simulink model "HighlyDynamicTrajectory_EuroGNC2022"  (R2018b)
settings: Solver=ode4  StartTime=0.0  StopTime=43.381  FixedStep=0.001  RelTol=1e-3
values from neighbouring files (symbols this model uses):
  airplane = conventionalAirplaneLoadParams(  	'params_conventional_airplane_EasyGlider' )    [init_HighlyDynamicTrajectory_EuroGNC2022.m]
  envir = envirLoadParams( 'envir_params_default', 'envir', 0 )    [init_HighlyDynamicTrajectory_EuroGNC2022.m]
  g = 9.81    [init_HighlyDynamicTrajectory_EuroGNC2022.m]
  inital_vel_vec = inital_velo * T    [init_HighlyDynamicTrajectory_EuroGNC2022.m]
  K_atti = ndiFeedbackGainPlace( -10*ones(3,1), 2/80 + 2/100 )    [init_HighlyDynamicTrajectory_EuroGNC2022.m]
  K_lateral = ndiFeedbackGainPlace( -0.75*ones(3,1), 0)    [init_HighlyDynamicTrajectory_EuroGNC2022.m]
  K_vertical = ndiFeedbackGainPlace(-2.0*ones(3,1), 0)    [init_HighlyDynamicTrajectory_EuroGNC2022.m]
  traj = trajFromWaypoints(traj, waypoints, degree, cycle)    [init_HighlyDynamicTrajectory_EuroGNC2022.m]
undefined symbols (not defined in the file or in its folder): aileron_left, aileron_right, alt_ground, atmosphere, ca, elevator, htp_trim, rudder, throttle, wind
libraries: actuators_lib x7, simulink x7, unit_conversions_lib x7, axes_transformation_lib x1, quat_lib x1, indi_lib x1, quatAttitudeController_lib x1, conventional_airplane_single_engine_lib x1, atmosphere_lib x1, sensors_lib x1, flightgear_visualization_lib x1
settings Model: Creator=Fgücker  LastModifiedBy=fabian

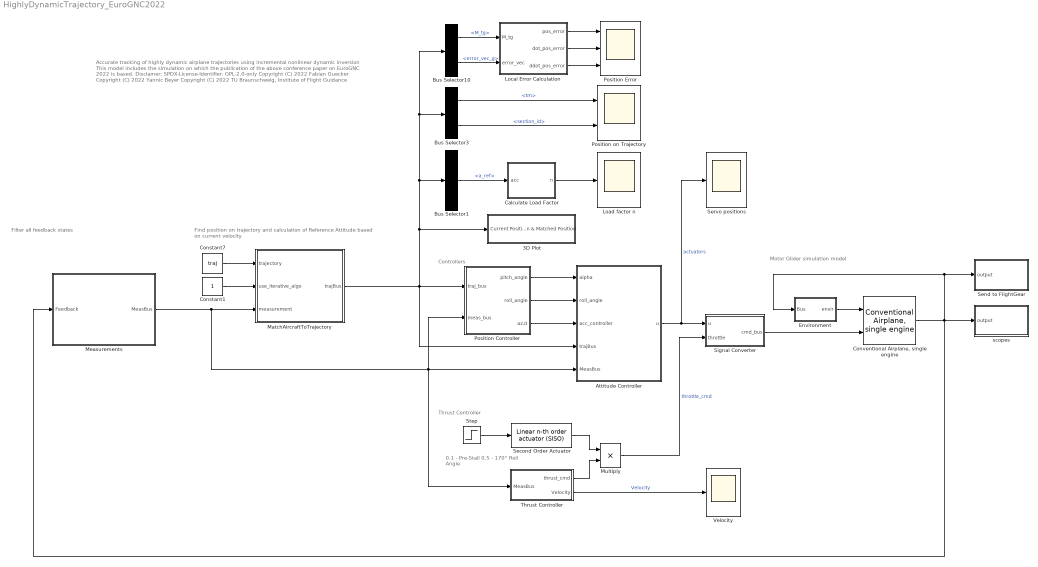
== system HighlyDynamicTrajectory_EuroGNC2022 ==
  note: Controllers
  note: 0.1 - Pre-Stall
      | 0.5 - 170° Roll Angle
  note: Accurate tracking of highly dynamic airplane
      | trajectories using incremental nonlinear dynamic
      | inversion
      |
      | This model includes the simulation on which the publication of the above conference paper on EuroGNC 2022 is based.
      |
      | Disclamer:
      | SPDX-License-Identifier: GPL-2.0-only
      |
      | Copyright (C) 2022 Fabian Guecker
      | Copyright (C) 2022 Yannic Beyer
      | Copyright (C) 2022 TU Braunschweig, Institute of Flight Guidance
  note: Thrust Controller
  note: Find position on trajectory and calculation
      | of Reference Attitude based on current velocity
  note: Filter all feedback states
  note: Motor Glider simulation model
  3D Plot : Subsystem
  Attitude Controller : Subsystem
  Bus Selector1 : BusSelector  OutputSignals=a_ref
  Bus Selector10 : BusSelector  OutputSignals=M_tg,error_vec_g
  Bus Selector3 : BusSelector  OutputSignals=tm,section_id
  Calculate Load Factor : Subsystem
  Constant1 : Constant
  Constant7 : Constant  Value=traj  OutDataTypeStr=Bus: trajectoryBus
  "Conventional Airplane, single engine" : conventional_airplane_single_engine_lib/Conventional Airplane, single engine  airplane=airplane
      settings: SourceProductName=LADAC
  Environment : Subsystem
  Load factor n : Scope
  Local Error Calculation : Subsystem
  MatchAircraftToTrajectory : Subsystem  SystemSampleTime=0.001
  Measurements : Subsystem  mask{omega0=50, D=0.55}
      mask prompts: omega0 "Omega - Filter"; D "Damping D - Filter"
  Multiply : Product
  Position Controller : Subsystem
  Position Error : Scope  NumInputPorts=3
  Position on Trajectory : Scope  NumInputPorts=2
  Second Order Actuator : actuators_lib/Linear n-th order actuator (SISO)  omega=10  order=2  output_order=1  use_inital_value=on
      settings: SourceProductName=LADAC
  Send to FlightGear : Subsystem
  Servo positions : Scope
  Signal Converter : Subsystem
  Step : Step  Time=26  Before=0.1  After=0.5  SampleTime=0
  Thrust Controller : Subsystem
  Velocity : Scope
  scopes : Subsystem
  wires:
  Measurements/1(MeasBus) -> Attitude Controller/5(MeasBus), Thrust Controller/1(MeasBus), Position Controller/2(meas_bus), MatchAircraftToTrajectory/3(measurement)
  Thrust Controller/1(thrust_cmd) -> Multiply/2
  Thrust Controller/2(Velocity) -> Velocity/1  "Velocity"
  Environment/1(envir) -> "Conventional Airplane, single engine"/1
  Local Error Calculation/3(ddot_pos_error) -> Position Error/3
  Local Error Calculation/2(dot_pos_error) -> Position Error/2
  Local Error Calculation/1(pos_error) -> Position Error/1
  Bus Selector10/2 -> Local Error Calculation/2(error_vec)  "<error_vec_g>"
  Multiply/1 -> Signal Converter/2(throttle)  "throttle_cmd"
  Constant7/1 -> MatchAircraftToTrajectory/1(trajectory)
  Bus Selector10/1 -> Local Error Calculation/1(M_tg)  "<M_tg>"
  Calculate Load Factor/1(n) -> Load factor n/1
  Bus Selector1/1 -> Calculate Load Factor/1(acc)  "<a_ref>"
  Bus Selector3/1 -> Position on Trajectory/1  "<tm>"
  Bus Selector3/2 -> Position on Trajectory/2  "<section_id>"
  Position Controller/1(pitch_angle) -> Attitude Controller/1(alpha)
  Position Controller/2(roll_angle) -> Attitude Controller/2(roll_angle)
  Constant1/1 -> MatchAircraftToTrajectory/2(use_iterative_algo)
  Position Controller/3(az,d) -> Attitude Controller/3(acc_controller)
  Step/1 -> Second Order Actuator/1
  Second Order Actuator/1 -> Multiply/1
  Signal Converter/1(cmd_bus) -> "Conventional Airplane, single engine"/2
  Attitude Controller/1(u) -> Servo positions/1, Signal Converter/1(u)  "actuators"
  MatchAircraftToTrajectory/1(trajBus) -> Bus Selector1/1, Bus Selector10/1, Bus Selector3/1, 3D Plot/1(Current Position & Matched Position), Position Controller/1(traj_bus), Attitude Controller/4(trajBus)
  "Conventional Airplane, single engine"/1 -> Measurements/1(Feedback), Environment/1(Bus), Send to FlightGear/1(output), scopes/1(output)

== system HighlyDynamicTrajectory_EuroGNC2022/3D Plot ==
  Current Position & Matched Position : Inport
  3D Graph : S-Function  LoadFcn=if exist('sfun3d','file'), sfun3d([],[],[],'LoadBlock'); end  FunctionName=sfun3d  Parameters=ax,T,np,cp,gd,ls,mk,mx,hd,tb  SFunctionDeploymentMode=off  EnableBusSupport=off  mask(3D Graph){np=2, ax=[-8 8 -8 8 -8 8]*20, mx=1e4, T=0.040, cp=[-1 -1 1]*35, gd=on, hd=off, tb=off, ls=-, mk=none}
      mask prompts: np "Number of moving points (lines)"; ax "Range: [xmin xmax  ymin ymax zmin zmax]"; mx "Max number of points in each line"; T "Sampling Time"; cp "Camera position (use [0 0 1] for 2D XY view)"; gd "Grid (on|off)"; hd "HeadMarkers (on|off)"; tb "Toolbar (on|off)"; ls "LineStyle"; mk "LineMarker"
      mask help:
      | This block plots the position of several points in the XYZ space. The input contains the coordinates of all the points (x1,y1,z1,x2,y2,z2,...).
      | The number of moving points (lines), the XYZ ranges, sampling time, camera position, and grid (among other things) can be set as mask parameters.
      settings: CopyFcn=if exist('sfun3d','file'), sfun3d([],[],[],'CopyBlock'); end  DeleteFcn=if exist('sfun3d','file'), sfun3d([],[],[],'DeleteBlock'); end  NameChangeFcn=if exist('sfun3d','file'), sfun3d([],[],[],'NameChange'); end
      mask Help:
      | This block plots the position of several points in the XYZ space. The input contains the coordinates of all the points (x1,y1,z1,x2,y2,z2,...).
      | The number of moving points (lines), the XYZ ranges, sampling time, camera position, and grid (among other things) can be set as mask parameters.
      mask TypeOptions ls: - | -- | : | -. | none
      mask TypeOptions mk: none | . | + | o | * | x | square | diamond | v | ^ | > | < | pentagram | hexagram
      mask Display: plot([.05 .95 .95 .05 .05],[.45 .45 .95 .95 .45], 0.5+cos(0:0.1:2*pi)*0.3,0.7+sin(0:0.1:2*pi)*0.2)
  Bus Selector5 : BusSelector  OutputSignals=s_g,position
  Gain19 : Gain  Gain=[1 1 -1]'
  Gain2 : Gain  Gain=[1 1 -1]'
  Mux : Mux  Inputs=2
  wires:
  Bus Selector5/2 -> Gain19/1  "<position>"
  Gain19/1 -> Mux/2
  Current Position & Matched Position/1 -> Bus Selector5/1
  Bus Selector5/1 -> Gain2/1  "<s_g>"
  Mux/1 -> 3D Graph/1
  Gain2/1 -> Mux/1

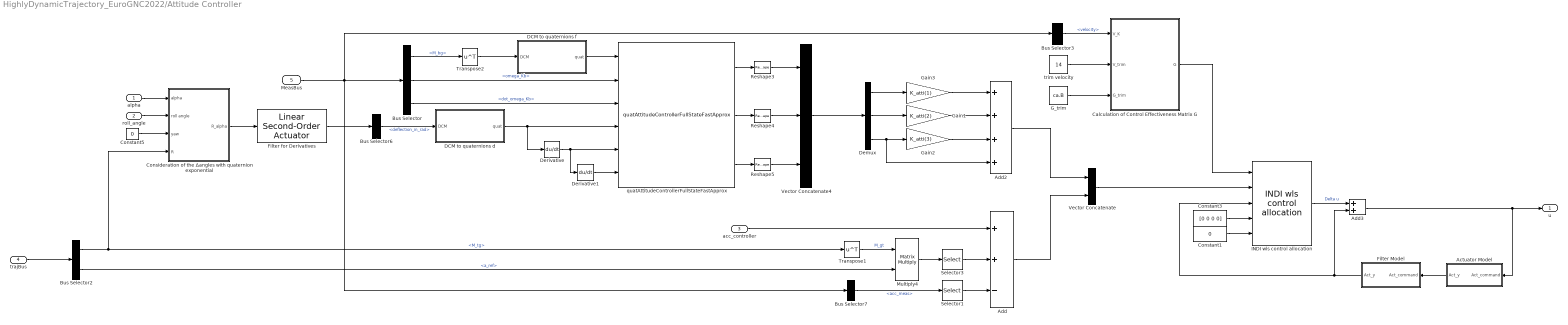
== system HighlyDynamicTrajectory_EuroGNC2022/Attitude Controller ==
  alpha : Inport
  roll_angle : Inport  Port=2
  acc_controller : Inport  Port=3
  trajBus : Inport  Port=4
  MeasBus : Inport  Port=5
  Actuator Model : Subsystem  mask{omega=[80 80 80 80]', d=1, A_0=[0 0 0 0]', dot_A_0=0, start_steady_state=off}
      mask prompts: omega "Natural frequency"; d "Damping ratio"; A_0 "Initial position"; dot_A_0 "Initial velocity"; start_steady_state "Start steady state"
  Add : Sum  Inputs=++-
  Add2 : Sum  Inputs=++++
  Add3 : Sum
  Bus Selector : BusSelector  OutputSignals=EKF.M_bg,EKF.omega_Kb,EKF.dot_omega_Kb
  Bus Selector2 : BusSelector  OutputSignals=M_tg,a_ref
  Bus Selector3 : BusSelector  OutputSignals=EKF.velocity
  Bus Selector6 : BusSelector  OutputSignals=deflection_in_rad
  Bus Selector7 : BusSelector  OutputSignals=accelerometer.acc_meas
  Calculation of Control Effectiveness Matrix G : Subsystem
  Consideration of the Δangles with quaternion exponential : Subsystem
  Constant1 : Constant  Value=0
  Constant3 : Constant  Value=[0 0 0 0]
  Constant5 : Constant  Value=0
  DCM to quaternions d : Subsystem
      mask DialogControl DescGroupVar Prompt: Get quaternions from DCM without discontinuities
      mask DialogControl DescTextVar Prompt: Look inside the block (and function) for more information.
  DCM to quaternions f : Subsystem
      mask DialogControl DescGroupVar Prompt: Get quaternions from DCM without discontinuities
      mask DialogControl DescTextVar Prompt: Look inside the block (and function) for more information.
  Demux : Demux  Outputs=3
  Derivative : Derivative
  Derivative1 : Derivative
  Filter Model : Subsystem  mask{omega=[50 50 50 50]', d=0.55, A_0=[0 0 0 0]', dot_A_0=0, start_steady_state=off}
      mask prompts: omega "Natural frequency"; d "Damping ratio"; A_0 "Initial position"; dot_A_0 "Initial velocity"; start_steady_state "Start steady state"
  Filter for Derivatives : actuators_lib/Linear Second-Order Actuator  omega=200  d=1  A_0=0  dot_A_0=0  start_steady_state=on
      settings: SourceProductName=LADAC
  G_trim : Constant  Value=ca.B
  Gain1 : Gain  Gain=K_atti(2)
  Gain2 : Gain  Gain=K_atti(3)
  Gain3 : Gain  Gain=K_atti(1)
  INDI wls control allocation : indi_lib/INDI wls control allocation  ca=ca
      settings: SourceProductName=LADAC
  Multiply4 : Product  Multiplication=Matrix(*)
  Reshape3 : Reshape  OutputDimensionality=Column vector (2-D)
  Reshape4 : Reshape  OutputDimensionality=Column vector (2-D)
  Reshape5 : Reshape  OutputDimensionality=Column vector (2-D)
  Selector1 : Selector  InputPortWidth=3  IndexOptions=Index vector (dialog)  Indices=[3]  OutputSizes=1
  Selector3 : Selector  InputPortWidth=3  IndexOptions=Index vector (dialog)  Indices=[3]  OutputSizes=1
  Transpose1 : Math  Operator=transpose  SaturateOnIntegerOverflow=on
  Transpose2 : Math  Operator=transpose  SaturateOnIntegerOverflow=on
  Vector Concatenate : Concatenate
  Vector Concatenate4 : Concatenate  NumInputs=3
  quatAttitudeControllerFullStateFastApprox : quatAttitudeController_lib/quatAttitudeControllerFullStateFastApprox  SystemSampleTime=-1
      settings: SourceProductName=LADAC
  trim velocity : Constant  Value=14
  u : Outport
  wires:
  Bus Selector/3 -> quatAttitudeControllerFullStateFastApprox/3  "<dot_omega_Kb>"
  Derivative1/1 -> quatAttitudeControllerFullStateFastApprox/6
  Filter for Derivatives/1 -> Bus Selector6/1
  Vector Concatenate4/1 -> Demux/1
  Bus Selector/2 -> quatAttitudeControllerFullStateFastApprox/2  "<omega_Kb>"
  Gain3/1 -> Add2/1
  Derivative/1 -> Derivative1/1, quatAttitudeControllerFullStateFastApprox/5
  Gain1/1 -> Add2/2
  Demux/3 -> Add2/4, Gain2/1
  Bus Selector/1 -> Transpose2/1  "<M_bg>"
  DCM to quaternions f/1(quat) -> quatAttitudeControllerFullStateFastApprox/1
  quatAttitudeControllerFullStateFastApprox/1 -> Reshape3/1
  Reshape3/1 -> Vector Concatenate4/1
  Reshape4/1 -> Vector Concatenate4/2
  Reshape5/1 -> Vector Concatenate4/3
  quatAttitudeControllerFullStateFastApprox/3 -> Reshape5/1
  Bus Selector6/1 -> DCM to quaternions d/1(DCM)  "<deflection_in_rad>"
  quatAttitudeControllerFullStateFastApprox/2 -> Reshape4/1
  roll_angle/1 -> Consideration of the Δangles with quaternion exponential/2(roll angle)
  Demux/1 -> Gain3/1
  Gain2/1 -> Add2/3
  Demux/2 -> Gain1/1
  DCM to quaternions d/1(quat) -> Derivative/1, quatAttitudeControllerFullStateFastApprox/4
  Transpose2/1 -> DCM to quaternions f/1(DCM)
  INDI wls control allocation/1 -> Add3/1  "Delta u"
  Bus Selector7/1 -> Selector1/1  "<acc_meas>"
  Transpose1/1 -> Multiply4/1  "M_gt"
  trajBus/1 -> Bus Selector2/1
  Multiply4/1 -> Selector3/1
  Bus Selector2/2 -> Multiply4/2  "<a_ref>"
  Selector1/1 -> Add/3
  Bus Selector2/1 -> Consideration of the Δangles with quaternion exponential/4(R), Transpose1/1  "<M_tg>"
  Vector Concatenate/1 -> INDI wls control allocation/2
  Add/1 -> Vector Concatenate/2
  acc_controller/1 -> Add/1
  Selector3/1 -> Add/2
  Add3/1 -> u/1, Actuator Model/1(Act_command)
  alpha/1 -> Consideration of the Δangles with quaternion exponential/1(alpha)
  MeasBus/1 -> Bus Selector3/1, Bus Selector7/1, Bus Selector/1
  Constant3/1 -> INDI wls control allocation/4
  Consideration of the Δangles with quaternion exponential/1(R_alpha) -> Filter for Derivatives/1
  Constant5/1 -> Consideration of the Δangles with quaternion exponential/3(yaw)
  Filter Model/1(Act_y) -> Add3/2, INDI wls control allocation/3
  Actuator Model/1(Act_y) -> Filter Model/1(Act_command)
  Bus Selector3/1 -> Calculation of Control Effectiveness Matrix G/1(V_K)  "<velocity>"
  trim velocity/1 -> Calculation of Control Effectiveness Matrix G/2(V_trim)
  G_trim/1 -> Calculation of Control Effectiveness Matrix G/3(G_trim)
  Calculation of Control Effectiveness Matrix G/1(G) -> INDI wls control allocation/1
  Constant1/1 -> INDI wls control allocation/5
  Add2/1 -> Vector Concatenate/1

== system HighlyDynamicTrajectory_EuroGNC2022/Calculate Load Factor ==
  acc : Inport
  Dot Product : DotProduct  InputSameDT=on  OutDataTypeStr=Inherit: Inherit via internal rule
  Gain7 : Gain  Gain=1/g
  Sqrt : Sqrt  SaturateOnIntegerOverflow=on
  n : Outport
  wires:
  Dot Product/1 -> Sqrt/1
  Sqrt/1 -> Gain7/1
  acc/1 -> Dot Product/1, Dot Product/2
  Gain7/1 -> n/1

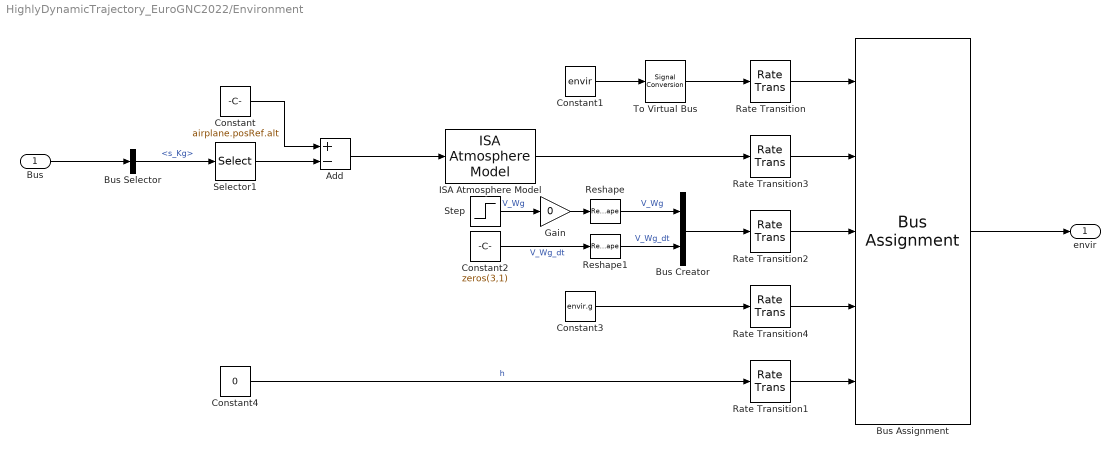
== system HighlyDynamicTrajectory_EuroGNC2022/Environment ==
  Bus : Inport
  Add : Sum  Inputs=+-
  Bus Assignment : BusAssignment  AssignedSignals=atmosphere,wind,g,alt_ground
  Bus Creator : BusCreator  Inputs=2
  Bus Selector : BusSelector  OutputSignals=rigidBodyBus.s_Kg
  Constant : Constant  Value=airplane.posRef.alt
  Constant1 : Constant  Value=envir  OutDataTypeStr=Bus: envirBus
  Constant2 : Constant  Value=zeros(3,1)
  Constant3 : Constant  Value=envir.g
  Constant4 : Constant  Value=0
  Gain : Gain  Gain=0
  ISA Atmosphere Model : atmosphere_lib/ISA Atmosphere Model  SystemSampleTime=-1
      settings: SourceProductName=LADAC
  Rate Transition{,1..4} (5 alike) : RateTransition
  Reshape : Reshape  OutputDimensionality=Column vector (2-D)
  Reshape1 : Reshape  OutputDimensionality=Column vector (2-D)
  Selector1 : Selector  InputPortWidth=3  IndexOptions=Index vector (dialog)  Indices=3  OutputSizes=1
  Step : Step  Time=3  After=[0;5;0]  SampleTime=0
  To Virtual Bus : SignalConversion  ConversionOutput=Virtual bus  OverrideOpt=off
  envir : Outport
  wires:
  Constant4/1 -> Rate Transition1/1  "h"
  Rate Transition2/1 -> Bus Assignment/3
  Rate Transition3/1 -> Bus Assignment/2
  Bus Assignment/1 -> envir/1
  Rate Transition/1 -> Bus Assignment/1
  ISA Atmosphere Model/1 -> Rate Transition3/1
  Step/1 -> Gain/1  "V_Wg"
  Rate Transition1/1 -> Bus Assignment/5
  Constant1/1 -> To Virtual Bus/1
  Bus/1 -> Bus Selector/1
  Bus Creator/1 -> Rate Transition2/1
  Constant2/1 -> Reshape1/1  "V_Wg_dt"
  Rate Transition4/1 -> Bus Assignment/4
  Constant3/1 -> Rate Transition4/1
  Gain/1 -> Reshape/1
  Constant/1 -> Add/1
  Add/1 -> ISA Atmosphere Model/1
  Selector1/1 -> Add/2
  To Virtual Bus/1 -> Rate Transition/1
  Reshape/1 -> Bus Creator/1  "V_Wg"
  Reshape1/1 -> Bus Creator/2  "V_Wg_dt"
  Bus Selector/1 -> Selector1/1  "<s_Kg>"

== system HighlyDynamicTrajectory_EuroGNC2022/Local Error Calculation ==
  M_tg : Inport
  error_vec : Inport  Port=2
  Derivative1 : Derivative
  Derivative2 : Derivative
  Multiply2 : Product  Multiplication=Matrix(*)
  Transpose : Math  Operator=transpose  SaturateOnIntegerOverflow=on
  pos_error : Outport
  dot_pos_error : Outport  Port=2
  ddot_pos_error : Outport  Port=3
  wires:
  error_vec/1 -> Multiply2/2
  Transpose/1 -> Multiply2/1
  M_tg/1 -> Transpose/1
  Derivative1/1 -> dot_pos_error/1, Derivative2/1
  Derivative2/1 -> ddot_pos_error/1
  Multiply2/1 -> Derivative1/1, pos_error/1

== system HighlyDynamicTrajectory_EuroGNC2022/MatchAircraftToTrajectory ==
  trajectory : Inport
  use_iterative_algo : Inport  Port=2
  measurement : Inport  Port=3
  Bus Creator : BusCreator  Inputs=8
  Bus Selector1 : BusSelector  OutputSignals=EKF.s_g,EKF.velocity
  Bus Selector3 : BusSelector  OutputSignals=EKF.s_g,EKF.velocity
  Constant : Constant  Value=[0; 0; -g]  VectorParams1D=off
  MATLAB Function6 : MATLAB Function  TreatAsAtomicUnit=on
  trajBus : Outport
  wires:
  Bus Selector3/1 -> MATLAB Function6/2(pos_ac)  "<s_g>"
  trajectory/1 -> MATLAB Function6/1(traj)  "trajectory"
  measurement/1 -> Bus Selector1/1, Bus Selector3/1
  Bus Creator/1 -> trajBus/1
  Bus Selector3/2 -> MATLAB Function6/3(vel)  "<velocity>"
  Constant/1 -> MATLAB Function6/4(acc_vec)
  use_iterative_algo/1 -> MATLAB Function6/5(use_iterative_algo)
  MATLAB Function6/1(pos) -> Bus Creator/1  "position"
  MATLAB Function6/2(error_vec) -> Bus Creator/2  "error_vec_g"
  MATLAB Function6/3(section_idx) -> Bus Creator/3  "section_id"
  MATLAB Function6/4(t) -> Bus Creator/4  "tm"
  MATLAB Function6/5(a_ref) -> Bus Creator/5  "a_ref"
  MATLAB Function6/6(M_tg) -> Bus Creator/6  "M_tg"
  Bus Selector1/1 -> Bus Creator/7  "<s_g>"
  Bus Selector1/2 -> Bus Creator/8  "<velocity>"

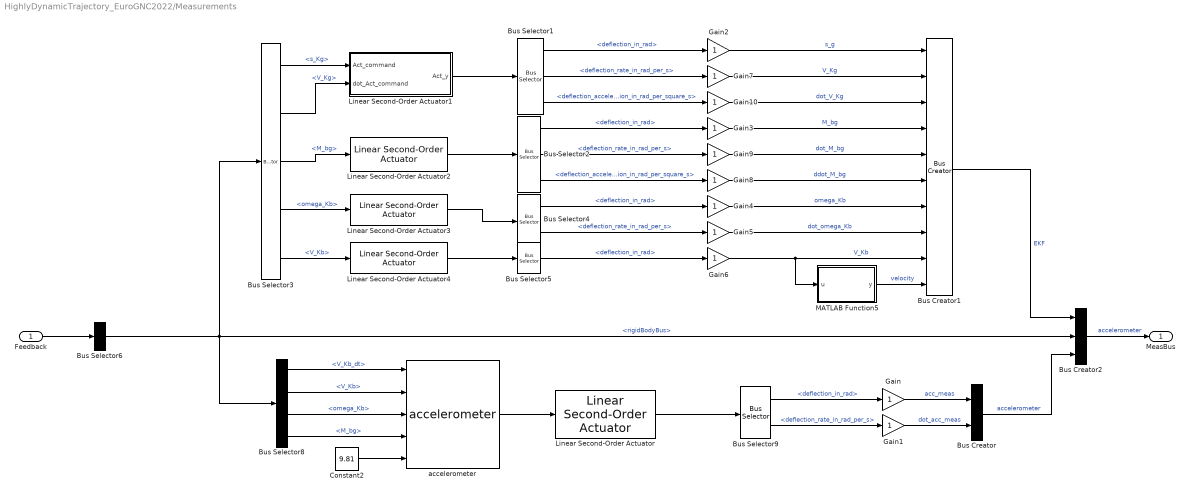
== system HighlyDynamicTrajectory_EuroGNC2022/Measurements ==
  Feedback : Inport
  Bus Creator : BusCreator  Inputs=2
  Bus Creator1 : BusCreator  Inputs=10
  Bus Creator2 : BusCreator  Inputs=3
  Bus Selector1 : BusSelector  OutputSignals=deflection_in_rad,deflection_rate_in_rad_per_s,deflection_acceleration_in_rad_per_square_s
  Bus Selector2 : BusSelector  OutputSignals=deflection_in_rad,deflection_rate_in_rad_per_s,deflection_acceleration_in_rad_per_square_s
  Bus Selector3 : BusSelector  OutputSignals=s_Kg,V_Kg,M_bg,omega_Kb,V_Kb
  Bus Selector4 : BusSelector  OutputSignals=deflection_in_rad,deflection_rate_in_rad_per_s
  Bus Selector5 : BusSelector  OutputSignals=deflection_in_rad
  Bus Selector6 : BusSelector  OutputSignals=rigidBodyBus
  Bus Selector8 : BusSelector  OutputSignals=V_Kb_dt,V_Kb,omega_Kb,M_bg
  Bus Selector9 : BusSelector  OutputSignals=deflection_in_rad,deflection_rate_in_rad_per_s
  Constant2 : Constant  Value=9.81
  Gain{,1..10} (11 alike) : Gain
  Linear Second-Order Actuator : actuators_lib/Linear Second-Order Actuator  omega=omega0  d=D  A_0=[0 0 -g]  dot_A_0=0  start_steady_state=off
      settings: SourceProductName=LADAC
  Linear Second-Order Actuator1 : Subsystem  mask{omega=omega0, d=D, A_0=0, dot_A_0=0}
      mask prompts: omega "Natural frequency"; d "Damping ratio"; A_0 "Initial position"; dot_A_0 "Initial velocity"
  Linear Second-Order Actuator2 : actuators_lib/Linear Second-Order Actuator  omega=omega0  d=D  A_0=0  dot_A_0=0  start_steady_state=on
      settings: SourceProductName=LADAC
  Linear Second-Order Actuator3 : actuators_lib/Linear Second-Order Actuator  omega=omega0  d=D  A_0=0  dot_A_0=0  start_steady_state=on
      settings: SourceProductName=LADAC
  Linear Second-Order Actuator4 : actuators_lib/Linear Second-Order Actuator  omega=omega0  d=D  A_0=0  dot_A_0=0  start_steady_state=on
      settings: SourceProductName=LADAC
  MATLAB Function5 : MATLAB Function  TreatAsAtomicUnit=on
  accelerometer : sensors_lib/accelerometer  SystemSampleTime=-1
  MeasBus : Outport
  wires:
  Bus Selector9/2 -> Gain1/1  "<deflection_rate_in_rad_per_s>"
  Bus Selector8/1 -> accelerometer/1  "<V_Kb_dt>"
  Linear Second-Order Actuator/1 -> Bus Selector9/1
  Bus Selector8/2 -> accelerometer/2  "<V_Kb>"
  Bus Selector8/3 -> accelerometer/3  "<omega_Kb>"
  Constant2/1 -> accelerometer/5
  Bus Selector8/4 -> accelerometer/4  "<M_bg>"
  accelerometer/1 -> Linear Second-Order Actuator/1
  Bus Selector9/1 -> Gain/1  "<deflection_in_rad>"
  Gain/1 -> Bus Creator/1  "acc_meas"
  Gain1/1 -> Bus Creator/2  "dot_acc_meas"
  Feedback/1 -> Bus Selector6/1
  Linear Second-Order Actuator1/1(Act_y) -> Bus Selector1/1
  Bus Selector3/1 -> Linear Second-Order Actuator1/1(Act_command)  "<s_Kg>"
  Bus Creator1/1 -> Bus Creator2/1  "EKF"
  Bus Creator2/1 -> MeasBus/1  "accelerometer"
  Bus Selector1/1 -> Gain2/1  "<deflection_in_rad>"
  Bus Selector3/3 -> Linear Second-Order Actuator2/1  "<M_bg>"
  Bus Selector3/4 -> Linear Second-Order Actuator3/1  "<omega_Kb>"
  Linear Second-Order Actuator2/1 -> Bus Selector2/1
  Linear Second-Order Actuator3/1 -> Bus Selector4/1
  Bus Selector4/2 -> Gain5/1  "<deflection_rate_in_rad_per_s>"
  Bus Selector4/1 -> Gain4/1  "<deflection_in_rad>"
  Bus Selector2/1 -> Gain3/1  "<deflection_in_rad>"
  Gain3/1 -> Bus Creator1/4  "M_bg"
  Gain4/1 -> Bus Creator1/7  "omega_Kb"
  Gain5/1 -> Bus Creator1/8  "dot_omega_Kb"
  Bus Selector3/5 -> Linear Second-Order Actuator4/1  "<V_Kb>"
  Linear Second-Order Actuator4/1 -> Bus Selector5/1
  Bus Selector5/1 -> Gain6/1  "<deflection_in_rad>"
  Gain6/1 -> MATLAB Function5/1(u), Bus Creator1/9  "V_Kb"
  MATLAB Function5/1(y) -> Bus Creator1/10  "velocity"
  Bus Creator/1 -> Bus Creator2/3  "accelerometer"
  Bus Selector1/2 -> Gain7/1  "<deflection_rate_in_rad_per_s>"
  Bus Selector3/2 -> Linear Second-Order Actuator1/2(dot_Act_command)  "<V_Kg>"
  Bus Selector2/2 -> Gain9/1  "<deflection_rate_in_rad_per_s>"
  Bus Selector2/3 -> Gain8/1  "<deflection_acceleration_in_rad_per_square_s>"
  Gain8/1 -> Bus Creator1/6  "ddot_M_bg"
  Gain9/1 -> Bus Creator1/5  "dot_M_bg"
  Bus Selector1/3 -> Gain10/1  "<deflection_acceleration_in_rad_per_square_s>"
  Gain2/1 -> Bus Creator1/1  "s_g"
  Gain7/1 -> Bus Creator1/2  "V_Kg"
  Gain10/1 -> Bus Creator1/3  "dot_V_Kg"
  Bus Selector6/1 -> Bus Selector3/1, Bus Creator2/2, Bus Selector8/1  "<rigidBodyBus>"

== system HighlyDynamicTrajectory_EuroGNC2022/Position Controller ==
  traj_bus : Inport
  meas_bus : Inport  Port=2
  Bus Selector : BusSelector  OutputSignals=EKF.velocity
  Error Calculation : Subsystem
  Lateral Controller : Subsystem
  Vertical Controller : Subsystem
  pitch_angle : Outport
  roll_angle : Outport  Port=2
  az,d : Outport  Port=3
  wires:
  Vertical Controller/1(pitch angle) -> pitch_angle/1
  Lateral Controller/1(roll_angle) -> roll_angle/1
  Vertical Controller/2(az_d) -> az,d/1
  Error Calculation/1("y_t, dot_y_t, ddot_y_t") -> Lateral Controller/1("y_t, dot_y_t, ddot_y_t")
  Error Calculation/2("z_t, dot_z_t, ddot_z_t") -> Vertical Controller/1("z_t, dot_z_t, ddot_z_t")
  traj_bus/1 -> Error Calculation/1(traj_bus)
  meas_bus/1 -> Bus Selector/1, Error Calculation/2(meas_bus)
  Bus Selector/1 -> Vertical Controller/2(V)  "<velocity>"

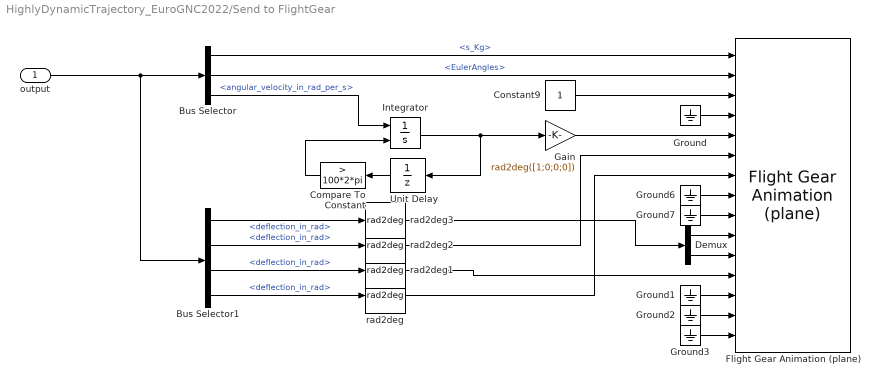
== system HighlyDynamicTrajectory_EuroGNC2022/Send to FlightGear ==
  output : Inport
  Bus Selector : BusSelector  OutputSignals=rigidBodyBus.s_Kg,rigidBodyBus.EulerAngles,actuatorBus.motorBus.angular_velocity_in_rad_per_s
  Bus Selector1 : BusSelector  OutputSignals=actuatorBus.aileronsBus.deflection_in_rad,actuatorBus.elevatorBus.deflection_in_rad,actuatorBus.rudderBus.deflection_in_rad,actuatorBus.htpTrimBus.deflection_in_rad
  Compare To Constant : simulink/Logic and Bit Operations/Compare To Constant  relop=>  const=100*2*pi  OutDataTypeStr=boolean
  Constant9 : Constant
  Demux : Demux  Outputs=2
  Flight Gear Animation (plane) : flightgear_visualization_lib/Flight Gear Animation (plane)  inital_lat=airplane.posRef.lat  inital_long=airplane.posRef.lon  inital_height=airplane.posRef.alt  remoteURL='127.0.0.1'  remotePort=5502
      settings: SourceProductName=LADAC
  Gain : Gain  Gain=rad2deg([1;0;0;0])
  Ground{,1..3,6..7} (6 alike) : Ground
  Integrator : Integrator  ExternalReset=rising
  Unit Delay : UnitDelay  SampleTime=-1
  rad2deg{,1..3} (4 alike) : unit_conversions_lib/rad2deg
      settings: SourceProductName=LADAC
  wires:
  Compare To Constant/1 -> Integrator/2
  Integrator/1 -> Unit Delay/1, Gain/1
  Bus Selector/1 -> Flight Gear Animation (plane)/1  "<s_Kg>"
  Bus Selector/2 -> Flight Gear Animation (plane)/2  "<EulerAngles>"
  Gain/1 -> Flight Gear Animation (plane)/5
  Constant9/1 -> Flight Gear Animation (plane)/3
  Unit Delay/1 -> Compare To Constant/1
  Ground/1 -> Flight Gear Animation (plane)/4
  Ground1/1 -> Flight Gear Animation (plane)/13
  Ground2/1 -> Flight Gear Animation (plane)/14
  Ground3/1 -> Flight Gear Animation (plane)/15
  output/1 -> Bus Selector1/1, Bus Selector/1
  Bus Selector/3 -> Integrator/1  "<angular_velocity_in_rad_per_s>"
  Bus Selector1/2 -> rad2deg2/1  "<deflection_in_rad>"
  Bus Selector1/4 -> rad2deg/1  "<deflection_in_rad>"
  Ground6/1 -> Flight Gear Animation (plane)/8
  Ground7/1 -> Flight Gear Animation (plane)/9
  Bus Selector1/3 -> rad2deg1/1  "<deflection_in_rad>"
  Bus Selector1/1 -> rad2deg3/1  "<deflection_in_rad>"
  Demux/1 -> Flight Gear Animation (plane)/10
  Demux/2 -> Flight Gear Animation (plane)/11
  rad2deg/1 -> Flight Gear Animation (plane)/7
  rad2deg1/1 -> Flight Gear Animation (plane)/12
  rad2deg2/1 -> Flight Gear Animation (plane)/6
  rad2deg3/1 -> Demux/1

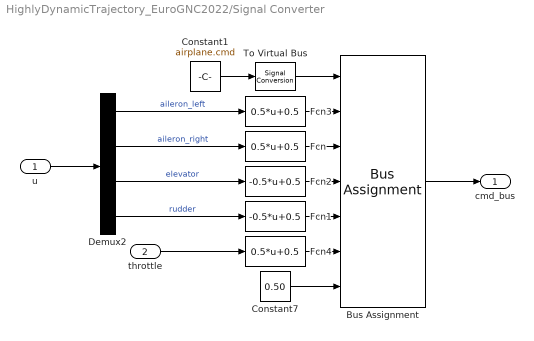
== system HighlyDynamicTrajectory_EuroGNC2022/Signal Converter ==
  u : Inport
  throttle : Inport  Port=2
  Bus Assignment : BusAssignment  AssignedSignals=aileron_left,aileron_right,elevator,rudder,throttle,htp_trim
  Constant1 : Constant  Value=airplane.cmd  OutDataTypeStr=Bus: cmdBus
  Constant7 : Constant  Value=0.50
  Demux2 : Demux
  Fcn : Fcn  Expr=0.5*u+0.5
  Fcn1 : Fcn  Expr=-0.5*u+0.5
  Fcn2 : Fcn  Expr=-0.5*u+0.5
  Fcn3 : Fcn  Expr=0.5*u+0.5
  Fcn4 : Fcn  Expr=0.5*u+0.5
  To Virtual Bus : SignalConversion  ConversionOutput=Virtual bus  OverrideOpt=off
  cmd_bus : Outport
  wires:
  Demux2/1 -> Fcn3/1  "aileron_left"
  Constant1/1 -> To Virtual Bus/1
  Demux2/4 -> Fcn1/1  "rudder"
  Fcn/1 -> Bus Assignment/3
  throttle/1 -> Fcn4/1
  Fcn3/1 -> Bus Assignment/2
  Demux2/3 -> Fcn2/1  "elevator"
  Fcn1/1 -> Bus Assignment/5
  Demux2/2 -> Fcn/1  "aileron_right"
  Fcn4/1 -> Bus Assignment/6
  u/1 -> Demux2/1
  To Virtual Bus/1 -> Bus Assignment/1
  Bus Assignment/1 -> cmd_bus/1
  Fcn2/1 -> Bus Assignment/4
  Constant7/1 -> Bus Assignment/7

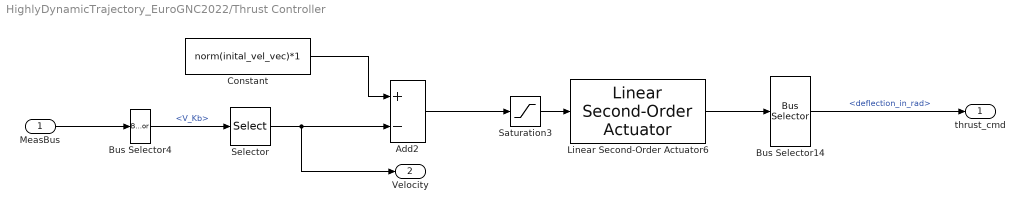
== system HighlyDynamicTrajectory_EuroGNC2022/Thrust Controller ==
  MeasBus : Inport
  Add2 : Sum  Inputs=+-
  Bus Selector14 : BusSelector  OutputSignals=deflection_in_rad
  Bus Selector4 : BusSelector  OutputSignals=EKF.V_Kb
  Constant : Constant  Value=norm(inital_vel_vec)*1
  Linear Second-Order Actuator6 : actuators_lib/Linear Second-Order Actuator  omega=20  d=1.5  A_0=0  dot_A_0=0  start_steady_state=off
      settings: SourceProductName=LADAC
  Saturation3 : Saturate  UpperLimit=10  LowerLimit=0
  Selector : Selector  InputPortWidth=3  IndexOptions=Index vector (dialog)  Indices=1  OutputSizes=1
  thrust_cmd : Outport
  Velocity : Outport  Port=2
  wires:
  Linear Second-Order Actuator6/1 -> Bus Selector14/1
  Selector/1 -> Velocity/1, Add2/2
  Add2/1 -> Saturation3/1
  Constant/1 -> Add2/1
  Bus Selector4/1 -> Selector/1  "<V_Kb>"
  MeasBus/1 -> Bus Selector4/1
  Saturation3/1 -> Linear Second-Order Actuator6/1
  Bus Selector14/1 -> thrust_cmd/1  "<deflection_in_rad>"

== system HighlyDynamicTrajectory_EuroGNC2022/scopes ==
  output : Inport
  Bus Selector : BusSelector  OutputSignals=rigidBodyBus,aeroBus,actuatorBus
  actuator scopes : Subsystem
  aero scopes : Subsystem
  rigid body scopes : Subsystem
  wires:
  Bus Selector/1 -> rigid body scopes/1(rigidBodyBus)  "<rigidBodyBus>"
  Bus Selector/2 -> aero scopes/1(aeroBus)  "<aeroBus>"
  output/1 -> Bus Selector/1
  Bus Selector/3 -> actuator scopes/1(actuatorBus)  "<actuatorBus>"

== system HighlyDynamicTrajectory_EuroGNC2022/Attitude Controller/Actuator Model ==
  Act_command : Inport
  2*d/omega : Gain  Gain=2*d./omega
  A : Integrator  InitialCondition=A_0  ContinuousStateAttributes='A'
  Sum2 : Sum  Inputs=|+-
  Sum3 : Sum  Inputs=|++
  dot_A : Integrator  InitialCondition=dot_A_0  ContinuousStateAttributes='dot_A'
  omega^2 : Gain  Gain=omega.^2
  Act_y : Outport
  wires:
  omega^2/1 -> dot_A/1  "deflection_acceleration_in_rad_per_square_s"
  Sum3/1 -> Sum2/2
  A/1 -> Act_y/1, Sum3/1  "deflection_in_rad"
  Sum2/1 -> omega^2/1
  Act_command/1 -> Sum2/1
  dot_A/1 -> A/1, 2*d/omega/1  "deflection_rate_in_rad_per_s"
  2*d/omega/1 -> Sum3/2

== system HighlyDynamicTrajectory_EuroGNC2022/Attitude Controller/Calculation of Control Effectiveness Matrix G ==
  V_K : Inport
  V_trim : Inport  Port=2
  G_trim : Inport  Port=3
  Dot Product : DotProduct  InputSameDT=on  OutDataTypeStr=Inherit: Inherit via internal rule
  Dot Product1 : DotProduct  InputSameDT=on  OutDataTypeStr=Inherit: Inherit via internal rule
  Multiply : Product  Inputs=*/*
  G : Outport
  wires:
  Dot Product1/1 -> Multiply/2
  G_trim/1 -> Multiply/3
  Multiply/1 -> G/1
  V_trim/1 -> Dot Product1/1, Dot Product1/2
  V_K/1 -> Dot Product/1, Dot Product/2
  Dot Product/1 -> Multiply/1

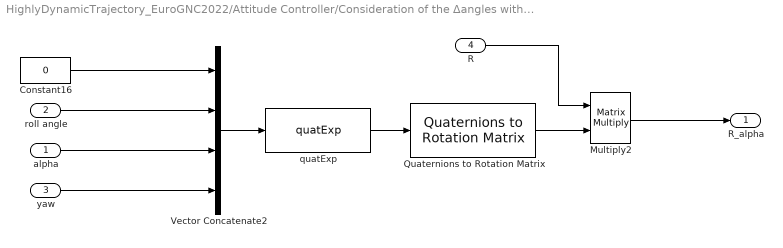
== system HighlyDynamicTrajectory_EuroGNC2022/Attitude Controller/Consideration of the Δangles with quaternion exponential ==
  alpha : Inport
  roll angle : Inport  Port=2
  yaw : Inport  Port=3
  R : Inport  Port=4
  Constant16 : Constant  Value=0
  Multiply2 : Product  Multiplication=Matrix(*)
  Quaternions to Rotation Matrix : axes_transformation_lib/Quaternions to Rotation Matrix  SystemSampleTime=-1
      settings: SourceProductName=LADAC
  Vector Concatenate2 : Concatenate  NumInputs=4
  quatExp : quat_lib/quatExp  SystemSampleTime=-1
      settings: SourceProductName=LADAC
  R_alpha : Outport
  wires:
  Multiply2/1 -> R_alpha/1
  Quaternions to Rotation Matrix/1 -> Multiply2/2
  Vector Concatenate2/1 -> quatExp/1
  R/1 -> Multiply2/1
  quatExp/1 -> Quaternions to Rotation Matrix/1
  alpha/1 -> Vector Concatenate2/3
  roll angle/1 -> Vector Concatenate2/2
  yaw/1 -> Vector Concatenate2/4
  Constant16/1 -> Vector Concatenate2/1

== system HighlyDynamicTrajectory_EuroGNC2022/Attitude Controller/DCM to quaternions d ==
  DCM : Inport
  DCM to quaternions : MATLAB Function  TreatAsAtomicUnit=on
  Delay : Delay  DelayLength=1  InitialConditionSource=Input port
      settings: InputPortMap=u0,p4
  MATLAB Function3 : MATLAB Function  TreatAsAtomicUnit=on
  quat : Outport
  wires:
  DCM to quaternions/1(q_bg) -> Delay/2
  MATLAB Function3/1(q_bg) -> quat/1, Delay/1  "q_bg"
  DCM/1 -> MATLAB Function3/1(M_bg), DCM to quaternions/1(M_bg)
  Delay/1 -> MATLAB Function3/2(last_q)

== system HighlyDynamicTrajectory_EuroGNC2022/Attitude Controller/DCM to quaternions f ==
  DCM : Inport
  DCM to quaternions : MATLAB Function  TreatAsAtomicUnit=on
  Delay : Delay  DelayLength=1  InitialConditionSource=Input port
      settings: InputPortMap=u0,p4
  MATLAB Function3 : MATLAB Function  TreatAsAtomicUnit=on
  quat : Outport
  wires:
  DCM to quaternions/1(q_bg) -> Delay/2
  MATLAB Function3/1(q_bg) -> quat/1, Delay/1  "q_bg"
  DCM/1 -> MATLAB Function3/1(M_bg), DCM to quaternions/1(M_bg)
  Delay/1 -> MATLAB Function3/2(last_q)

== system HighlyDynamicTrajectory_EuroGNC2022/Attitude Controller/Filter Model ==
  Act_command : Inport
  2*d/omega : Gain  Gain=2*d./omega
  A : Integrator  InitialCondition=A_0  ContinuousStateAttributes='A'
  Sum2 : Sum  Inputs=|+-
  Sum3 : Sum  Inputs=|++
  dot_A : Integrator  InitialCondition=dot_A_0  ContinuousStateAttributes='dot_A'
  omega^2 : Gain  Gain=omega.^2
  Act_y : Outport
  wires:
  omega^2/1 -> dot_A/1  "deflection_acceleration_in_rad_per_square_s"
  Sum3/1 -> Sum2/2
  A/1 -> Act_y/1, Sum3/1  "deflection_in_rad"
  Sum2/1 -> omega^2/1
  Act_command/1 -> Sum2/1
  dot_A/1 -> A/1, 2*d/omega/1  "deflection_rate_in_rad_per_s"
  2*d/omega/1 -> Sum3/2

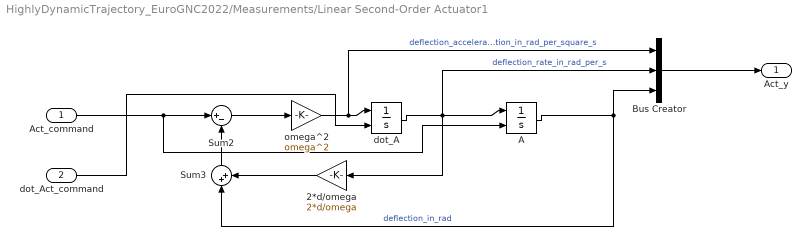
== system HighlyDynamicTrajectory_EuroGNC2022/Measurements/Linear Second-Order Actuator1 ==
  Act_command : Inport
  dot_Act_command : Inport  Port=2
  2*d/omega : Gain  Gain=2*d/omega
  A : Integrator  InitialConditionSource=external  InitialCondition=A_0  ContinuousStateAttributes='A'
  Bus Creator : BusCreator  Inputs=3
  Sum2 : Sum  Inputs=|+-
  Sum3 : Sum  Inputs=|++
  dot_A : Integrator  InitialConditionSource=external  InitialCondition=dot_A_0  ContinuousStateAttributes='dot_A'
  omega^2 : Gain  Gain=omega^2
  Act_y : Outport
  wires:
  Bus Creator/1 -> Act_y/1
  omega^2/1 -> dot_A/1, Bus Creator/1  "deflection_acceleration_in_rad_per_square_s"
  Sum3/1 -> Sum2/2
  A/1 -> Sum3/1, Bus Creator/3  "deflection_in_rad"
  Sum2/1 -> omega^2/1
  Act_command/1 -> A/2, Sum2/1
  dot_A/1 -> A/1, Bus Creator/2, 2*d/omega/1  "deflection_rate_in_rad_per_s"
  2*d/omega/1 -> Sum3/2
  dot_Act_command/1 -> dot_A/2

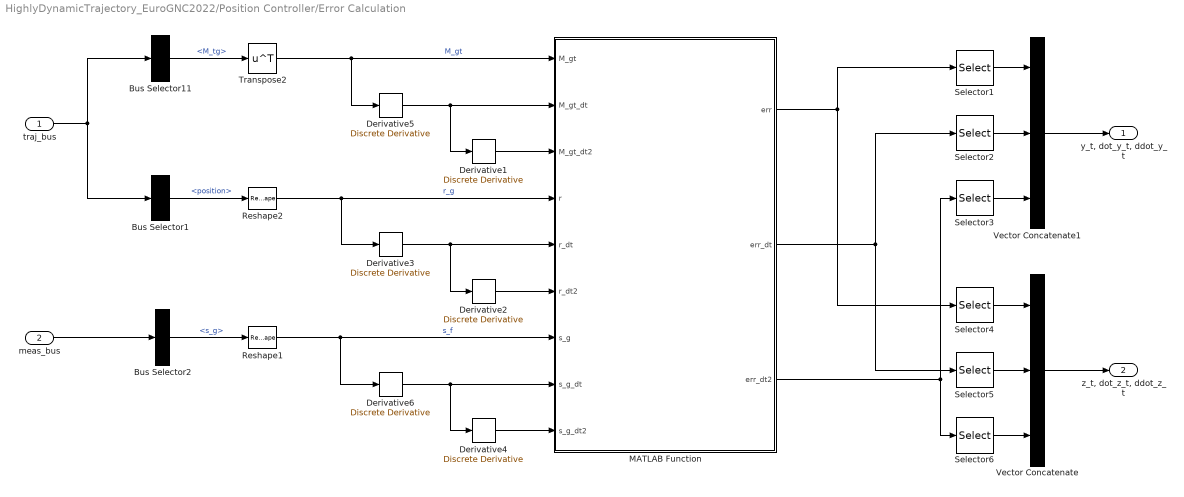
== system HighlyDynamicTrajectory_EuroGNC2022/Position Controller/Error Calculation ==
  traj_bus : Inport
  meas_bus : Inport  Port=2
  Bus Selector1 : BusSelector  OutputSignals=position
  Bus Selector11 : BusSelector  OutputSignals=M_tg
  Bus Selector2 : BusSelector  OutputSignals=EKF.s_g
  Derivative{1..6} (6 alike) : simulink/Discrete/Discrete Derivative  gainval=1.0  ICPrevScaledInput=0.0  OutMin=[]  OutMax=[]  OutDataType=fixdt(1, 16)  OutScaling=2^-10  DoSatur=off
  MATLAB Function : MATLAB Function  TreatAsAtomicUnit=on
  Reshape1 : Reshape  OutputDimensionality=Column vector (2-D)
  Reshape2 : Reshape  OutputDimensionality=Column vector (2-D)
  Selector1 : Selector  InputPortWidth=3  IndexOptions=Index vector (dialog)  Indices=2  OutputSizes=1
  Selector2 : Selector  InputPortWidth=3  IndexOptions=Index vector (dialog)  Indices=2  OutputSizes=1
  Selector3 : Selector  InputPortWidth=3  IndexOptions=Index vector (dialog)  Indices=2  OutputSizes=1
  Selector4 : Selector  InputPortWidth=3  IndexOptions=Index vector (dialog)  Indices=3  OutputSizes=1
  Selector5 : Selector  InputPortWidth=3  IndexOptions=Index vector (dialog)  Indices=3  OutputSizes=1
  Selector6 : Selector  InputPortWidth=3  IndexOptions=Index vector (dialog)  Indices=3  OutputSizes=1
  Transpose2 : Math  Operator=transpose  SaturateOnIntegerOverflow=on
  Vector Concatenate : Concatenate  NumInputs=3
  Vector Concatenate1 : Concatenate  NumInputs=3
  "y_t, dot_y_t, ddot_y_t" : Outport
  "z_t, dot_z_t, ddot_z_t" : Outport  Port=2
  wires:
  Derivative1/1 -> MATLAB Function/3(M_gt_dt2)
  Bus Selector11/1 -> Transpose2/1  "<M_tg>"
  MATLAB Function/1(err) -> Selector4/1, Selector1/1
  Derivative5/1 -> MATLAB Function/2(M_gt_dt), Derivative1/1
  MATLAB Function/3(err_dt2) -> Selector6/1, Selector3/1
  MATLAB Function/2(err_dt) -> Selector5/1, Selector2/1
  Selector3/1 -> Vector Concatenate1/3
  Selector1/1 -> Vector Concatenate1/1
  Selector2/1 -> Vector Concatenate1/2
  Selector6/1 -> Vector Concatenate/3
  Selector5/1 -> Vector Concatenate/2
  Selector4/1 -> Vector Concatenate/1
  Vector Concatenate/1 -> "z_t, dot_z_t, ddot_z_t"/1
  Vector Concatenate1/1 -> "y_t, dot_y_t, ddot_y_t"/1
  Transpose2/1 -> Derivative5/1, MATLAB Function/1(M_gt)  "M_gt"
  traj_bus/1 -> Bus Selector11/1, Bus Selector1/1
  Bus Selector1/1 -> Reshape2/1  "<position>"
  Reshape2/1 -> Derivative3/1, MATLAB Function/4(r)  "r_g"
  meas_bus/1 -> Bus Selector2/1
  Bus Selector2/1 -> Reshape1/1  "<s_g>"
  Derivative3/1 -> MATLAB Function/5(r_dt), Derivative2/1
  Derivative2/1 -> MATLAB Function/6(r_dt2)
  Derivative6/1 -> MATLAB Function/8(s_g_dt), Derivative4/1
  Derivative4/1 -> MATLAB Function/9(s_g_dt2)
  Reshape1/1 -> Derivative6/1, MATLAB Function/7(s_g)  "s_f"

== system HighlyDynamicTrajectory_EuroGNC2022/Position Controller/Lateral Controller ==
  note: Integration
  note: Control effectiveness
  "y_t, dot_y_t, ddot_y_t" : Inport
  Constant : Constant  Value=-1
  Constant1 : Constant  Value=9.81
  Divide : Product  Inputs=*/
  Gain12 : Gain  Gain=K_lateral  Multiplication=Matrix(K*u)
  Integrator1 : Integrator  LimitOutput=on  UpperSaturationLimit=45/57.3  LowerSaturationLimit=-45/57.3
  Multiply : Product
  Saturation : Saturate  UpperLimit=[20 inf inf]  LowerLimit=-[20 inf inf]
  Saturation1 : Saturate  UpperLimit=5  LowerLimit=-5
  roll_angle : Outport  PortDimensions=1
  wires:
  Constant/1 -> Divide/1
  Saturation/1 -> Gain12/1
  Gain12/1 -> Multiply/2
  Divide/1 -> Multiply/1
  Integrator1/1 -> roll_angle/1
  Constant1/1 -> Divide/2
  "y_t, dot_y_t, ddot_y_t"/1 -> Saturation/1
  Saturation1/1 -> Integrator1/1
  Multiply/1 -> Saturation1/1

== system HighlyDynamicTrajectory_EuroGNC2022/Position Controller/Vertical Controller ==
  note: Control effectiveness
  "z_t, dot_z_t, ddot_z_t" : Inport
  V : Inport  Port=2  PortDimensions=1
  Constant1 : Constant
  Divide1 : Product  Inputs=*/
  Gain1 : Gain  Gain=K_vertical  Multiplication=Matrix(K*u)
  "Limit Angle, Rate, Anti-Windup" : Subsystem
  Multiply1 : Product
  Saturation : Saturate  UpperLimit=30  LowerLimit=5
  pitch angle : Outport  PortDimensions=1
  az_d : Outport  Port=2
  wires:
  Gain1/1 -> Multiply1/2
  V/1 -> Saturation/1
  Constant1/1 -> Divide1/1
  Divide1/1 -> Multiply1/1
  "Limit Angle, Rate, Anti-Windup"/1(Out) -> pitch angle/1
  Saturation/1 -> Divide1/2
  Multiply1/1 -> "Limit Angle, Rate, Anti-Windup"/1(In1)
  "Limit Angle, Rate, Anti-Windup"/2(ddH) -> az_d/1
  "z_t, dot_z_t, ddot_z_t"/1 -> Gain1/1

== system HighlyDynamicTrajectory_EuroGNC2022/scopes/actuator scopes ==
  actuatorBus : Inport
  Bus Selector : BusSelector  OutputSignals=aileronsBus.deflection_in_rad,elevatorBus.deflection_in_rad,rudderBus.deflection_in_rad,htpTrimBus.deflection_in_rad,motorBus.angular_velocity_in_rad_per_s
  ailerons : Scope
  elevator : Scope
  htpTrim : Scope
  motor : Scope
  rudder : Scope
  wires:
  actuatorBus/1 -> Bus Selector/1
  Bus Selector/1 -> ailerons/1  "<deflection_in_rad>"
  Bus Selector/2 -> elevator/1  "<deflection_in_rad>"
  Bus Selector/3 -> rudder/1  "<deflection_in_rad>"
  Bus Selector/4 -> htpTrim/1  "<deflection_in_rad>"
  Bus Selector/5 -> motor/1  "<angular_velocity_in_rad_per_s>"

== system HighlyDynamicTrajectory_EuroGNC2022/scopes/aero scopes ==
  aeroBus : Inport
  Bus Selector : BusSelector  OutputSignals=aeroMainWing,aeroHtp,aerVtp,aeroFuse
  Bus Selector1 : BusSelector  OutputSignals=R_Ab,Q_Ab
  Scope : Scope
  Scope1 : Scope
  Subsystem : Subsystem
  Subsystem1 : Subsystem
  Subsystem2 : Subsystem
  wires:
  aeroBus/1 -> Bus Selector/1
  Bus Selector/1 -> Subsystem/1(In1)  "<aeroMainWing>"
  Bus Selector/2 -> Subsystem1/1(In1)  "<aeroHtp>"
  Bus Selector/3 -> Subsystem2/1(In1)  "<aerVtp>"
  Bus Selector/4 -> Bus Selector1/1  "<aeroFuse>"
  Bus Selector1/1 -> Scope/1  "<R_Ab>"
  Bus Selector1/2 -> Scope1/1  "<Q_Ab>"

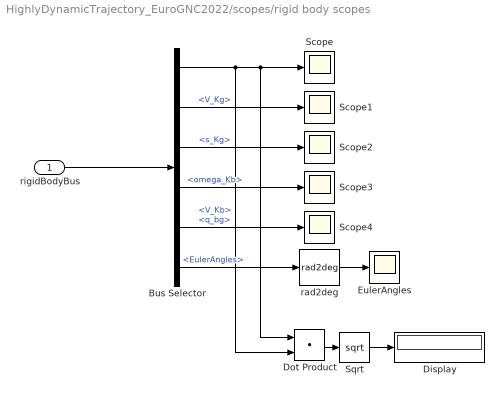
== system HighlyDynamicTrajectory_EuroGNC2022/scopes/rigid body scopes ==
  rigidBodyBus : Inport
  Bus Selector : BusSelector  OutputSignals=V_Kb,V_Kg,s_Kg,omega_Kb,q_bg,EulerAngles
  Display : Display
  Dot Product : DotProduct  InputSameDT=on  OutDataTypeStr=Inherit: Inherit via internal rule
  EulerAngles : Scope
  Scope{,1..4} (5 alike) : Scope
  Sqrt : Sqrt  SaturateOnIntegerOverflow=on
  rad2deg : unit_conversions_lib/rad2deg
      settings: SourceProductName=LADAC
  wires:
  rigidBodyBus/1 -> Bus Selector/1
  Bus Selector/1 -> Dot Product/2, Dot Product/1, Scope/1  "<V_Kb>"
  Bus Selector/2 -> Scope1/1  "<V_Kg>"
  Bus Selector/3 -> Scope2/1  "<s_Kg>"
  Bus Selector/4 -> Scope3/1  "<omega_Kb>"
  Bus Selector/5 -> Scope4/1  "<q_bg>"
  Bus Selector/6 -> rad2deg/1  "<EulerAngles>"
  Dot Product/1 -> Sqrt/1
  Sqrt/1 -> Display/1
  rad2deg/1 -> EulerAngles/1

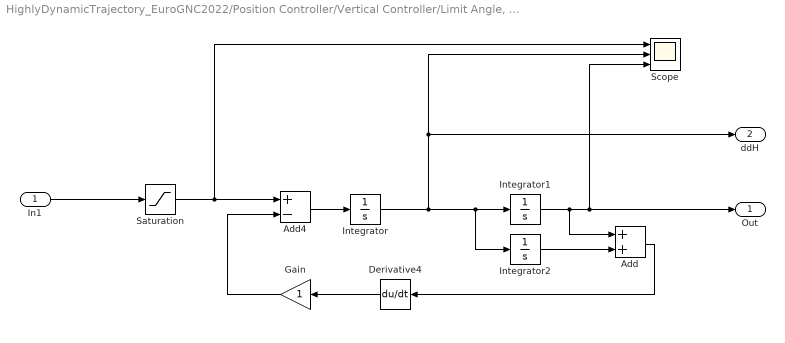
== system HighlyDynamicTrajectory_EuroGNC2022/Position Controller/Vertical Controller/Limit Angle, Rate, Anti-Windup ==
  In1 : Inport
  Add : Sum
  Add4 : Sum  Inputs=+-
  Derivative4 : Derivative
  Gain : Gain
  Integrator : Integrator  LimitOutput=on  UpperSaturationLimit=0.8  LowerSaturationLimit=-0.8
  Integrator1 : Integrator  LimitOutput=on  UpperSaturationLimit=45/57.3  LowerSaturationLimit=-45/57.3
  Integrator2 : Integrator
  Saturation : Saturate  UpperLimit=5  LowerLimit=-5
  Scope : Scope  NumInputPorts=3
  Out : Outport
  ddH : Outport  Port=2
  wires:
  Gain/1 -> Add4/2
  Integrator1/1 -> Scope/3, Out/1, Add/1
  Derivative4/1 -> Gain/1
  Add/1 -> Derivative4/1
  In1/1 -> Saturation/1
  Add4/1 -> Integrator/1
  Integrator2/1 -> Add/2
  Integrator/1 -> Scope/2, ddH/1, Integrator2/1, Integrator1/1
  Saturation/1 -> Scope/1, Add4/1

== system HighlyDynamicTrajectory_EuroGNC2022/scopes/aero scopes/Subsystem ==
  In1 : Inport
  Bus Selector : BusSelector  OutputSignals=aeroAxes.alpha_M_P,aeroAxes.beta_M_P,aeroAxes.q_P,dynamicsBody.R_Ab,dynamicsBody.Q_Ab,dynamicsBody.xyz_np_b,dynamicsBody.C_m_camber_np_b
  Scope{,1..6} (7 alike) : Scope
  rad2deg : unit_conversions_lib/rad2deg
      settings: SourceProductName=LADAC
  wires:
  In1/1 -> Bus Selector/1
  Bus Selector/1 -> rad2deg/1  "<alpha_M_P>"
  Bus Selector/3 -> Scope2/1  "<q_P>"
  Bus Selector/2 -> Scope1/1  "<beta_M_P>"
  Bus Selector/4 -> Scope3/1  "<R_Ab>"
  Bus Selector/5 -> Scope4/1  "<Q_Ab>"
  Bus Selector/6 -> Scope5/1  "<xyz_np_b>"
  Bus Selector/7 -> Scope6/1  "<C_m_camber_np_b>"
  rad2deg/1 -> Scope/1

== system HighlyDynamicTrajectory_EuroGNC2022/scopes/aero scopes/Subsystem1 ==
  In1 : Inport
  Bus Selector : BusSelector  OutputSignals=aeroAxes.alpha_M_P,aeroAxes.beta_M_P,aeroAxes.q_P,dynamicsBody.R_Ab,dynamicsBody.Q_Ab
  Scope{,1..4} (5 alike) : Scope
  rad2deg : unit_conversions_lib/rad2deg
      settings: SourceProductName=LADAC
  wires:
  Bus Selector/5 -> Scope4/1  "<Q_Ab>"
  Bus Selector/4 -> Scope3/1  "<R_Ab>"
  Bus Selector/2 -> Scope1/1  "<beta_M_P>"
  Bus Selector/3 -> Scope2/1  "<q_P>"
  Bus Selector/1 -> rad2deg/1  "<alpha_M_P>"
  In1/1 -> Bus Selector/1
  rad2deg/1 -> Scope/1

== system HighlyDynamicTrajectory_EuroGNC2022/scopes/aero scopes/Subsystem2 ==
  In1 : Inport
  Bus Selector : BusSelector  OutputSignals=aeroAxes.alpha_M_P,aeroAxes.beta_M_P,aeroAxes.q_P,dynamicsBody.R_Ab,dynamicsBody.Q_Ab
  Scope{,1..4} (5 alike) : Scope
  wires:
  In1/1 -> Bus Selector/1
  Bus Selector/1 -> Scope/1  "<alpha_M_P>"
  Bus Selector/3 -> Scope2/1  "<q_P>"
  Bus Selector/2 -> Scope1/1  "<beta_M_P>"
  Bus Selector/4 -> Scope3/1  "<R_Ab>"
  Bus Selector/5 -> Scope4/1  "<Q_Ab>"

== matlab function HighlyDynamicTrajectory_EuroGNC2022/MatchAircraftToTrajectory/MATLAB Function6 ==
  data: pos output; error_vec output; traj input; pos_ac input; section_idx output; t output; vel input; acc_vec input; use_iterative_algo input; a_ref output; M_tg output
function [pos, error_vec, section_idx, t, a_ref, M_tg]  = GetMatch(traj, pos_ac, vel, acc_vec, use_iterative_algo)

section_idx = 1;
t = 0;

if use_iterative_algo 
     [section_idx, ~, t] = trajGetMatchEnhanced(traj, pos_ac, section_idx);
else
     [section_idx, ~, t] = trajGetMatch(traj, pos_ac, section_idx);
end

traj_section = trajGetSection(traj, section_idx);

pos = trajSectionGetPos(traj_section, t);

error_vec = (pos - pos_ac);

[T, B, N, kappa, ~] = trajSectionGetFrenetSerretWithAcceleration(traj_section, vel, acc_vec, t);

% Calculate path acceleration
a_ref = (kappa * vel^2) * N;

M_tg = [T, B, -N];


end

== matlab function HighlyDynamicTrajectory_EuroGNC2022/Attitude Controller/DCM to quaternions d/DCM to quaternions ==
  data: M_bg input; q_bg output
function q_bg  = fcn( M_bg ) %#codegen
q_bg  = rotm2quat( M_bg );

== matlab function HighlyDynamicTrajectory_EuroGNC2022/Attitude Controller/DCM to quaternions d/MATLAB Function3 ==
  data: M_bg input; q_bg output; last_q input
function q_bg  = dcm2QuatCont( M_bg, last_q )

% dcm2Quat computes the quaternion (q_bg) from the direction cosine matrix
% (DCM) so that there are no discontinuities.
%   The quaternion is used to represent the attitude of the body
%   relative to the earth. It can be computed from the DCM. However, there
%   exist two solutions with reversed signs. This function avoids steps
%   which can be important for controllers.
% 
% Literature:
%   [1] Wu, J. (2018). Optimal Continuous Unit Quaternions from Rotation
%       Matrices. Journal of Guidance, Control and Dynamics.
% 
% Inputs:
%   M_bg            direction cosine matrix (with 3x3 elements) from NED
%                   frame (g) to body frame (b).
% 
% Outputs:
%   q_bg            quaternion vector with 4 elements and euclean norm of 1
% 
% See also: dcm2Quat
% 

% Disclamer:
%   SPDX-License-Identifier: GPL-2.0-only
% 
%   Copyright (C) 2020-2022 Yannic Beyer
%   Copyright (C) 2022 TU Braunschweig, Institute of Flight Guidance
% *************************************************************************

% get quaternions (with discontinuities)

%q_bg = dcm2Quat( M_bg );
q_bg = rotm2quat(M_bg)';

% remove discontinuities
q_bg = sign(q_bg' * last_q) * q_bg;


end

== matlab function HighlyDynamicTrajectory_EuroGNC2022/Attitude Controller/DCM to quaternions f/DCM to quaternions ==
  data: M_bg input; q_bg output
function q_bg  = fcn( M_bg ) %#codegen
q_bg  = rotm2quat( M_bg );

== matlab function HighlyDynamicTrajectory_EuroGNC2022/Attitude Controller/DCM to quaternions f/MATLAB Function3 ==
  data: M_bg input; q_bg output; last_q input
function q_bg  = dcm2QuatCont( M_bg, last_q )

% dcm2Quat computes the quaternion (q_bg) from the direction cosine matrix
% (DCM) so that there are no discontinuities.
%   The quaternion is used to represent the attitude of the body
%   relative to the earth. It can be computed from the DCM. However, there
%   exist two solutions with reversed signs. This function avoids steps
%   which can be important for controllers.
% 
% Literature:
%   [1] Wu, J. (2018). Optimal Continuous Unit Quaternions from Rotation
%       Matrices. Journal of Guidance, Control and Dynamics.
% 
% Inputs:
%   M_bg            direction cosine matrix (with 3x3 elements) from NED
%                   frame (g) to body frame (b).
% 
% Outputs:
%   q_bg            quaternion vector with 4 elements and euclean norm of 1
% 
% See also: dcm2Quat
% 

% Disclamer:
%   SPDX-License-Identifier: GPL-2.0-only
% 
%   Copyright (C) 2020-2022 Yannic Beyer
%   Copyright (C) 2022 TU Braunschweig, Institute of Flight Guidance
% *************************************************************************

% get quaternions (with discontinuities)

%q_bg = dcm2Quat( M_bg );
q_bg = rotm2quat(M_bg)';

% remove discontinuities
q_bg = sign(q_bg' * last_q) * q_bg;


end

== matlab function HighlyDynamicTrajectory_EuroGNC2022/Measurements/MATLAB Function5 ==
  data: u input; y output
function y = fcn(u)

y = norm(u);

== matlab function HighlyDynamicTrajectory_EuroGNC2022/Position Controller/Error Calculation/MATLAB Function ==
  data: M_gt input; err output; M_gt_dt input; M_gt_dt2 input; r input; r_dt input; r_dt2 input; s_g input; s_g_dt input; s_g_dt2 input; err_dt output; err_dt2 output
function [err, err_dt, err_dt2] = fcn(M_gt, M_gt_dt, M_gt_dt2, r, r_dt, r_dt2, s_g, s_g_dt, s_g_dt2)

err = M_gt * (r - s_g);
err_dt = M_gt * (r_dt - s_g_dt) + M_gt_dt * (r - s_g);
err_dt2 = M_gt*(r_dt2 - s_g_dt2) + 2*M_gt_dt*(r_dt - s_g_dt) + M_gt_dt2*(r - s_g);

end
